simulink model "MPCtest1"  (Simulink 10.1)
settings: Solver=VariableStepAuto  StartTime=0.0  StopTime=30  RelTol=1e-3
libraries: Solver_SF x1, sldrtlib x1, simulink x1
settings Model: Creator=27286  LastModifiedBy=27286
settings DataIOCC: SaveFormat=Dataset  ReturnWorkspaceOutputs=on
settings OptimizationCC: LifeSpan=auto
settings DebuggingCC: UnderspecifiedInitializationDetection=Simplified  MergeDetectMultiDrivingBlocksExec=error  SFUnexpectedBacktrackingDiag=error  SFNoUnconditionalDefaultTransitionDiag=error  SFExecutionAtInitializationDiag=warning  ArithmeticOperatorsInVariantConditions=error
settings HardwareCC: ProdBitPerPointer=64  ProdBitPerSizeT=64  ProdBitPerPtrDiffT=64  ProdLargestAtomicFloat=Float  ProdIntDivRoundTo=Zero  ProdEndianess=LittleEndian  ProdWordSize=64  ProdHWDeviceType=Intel->x86-64 (Windows64)
settings ModelReferenceCC: PropagateSignalLabelsOutOfModel=on
settings SFSimCC: SimUseLocalCustomCode=on  CustomCodeUndefinedFunction=FilterOut
settings RTWCC: RTWUseLocalCustomCode=on
settings CodeAppCC: StateflowObjectComments=off
settings GRTTargetCC: TargetLangStandard=C99 (ISO)  CombineOutputUpdateFcns=on  GRTInterface=off
settings ConfigComp: CovMetricSettings=dwe  CovHtmlReporting=off  CovSaveCumulativeToWorkspaceVar=off  CovSaveSingleToWorkspaceVar=off  CovExternalEMLEnable=on

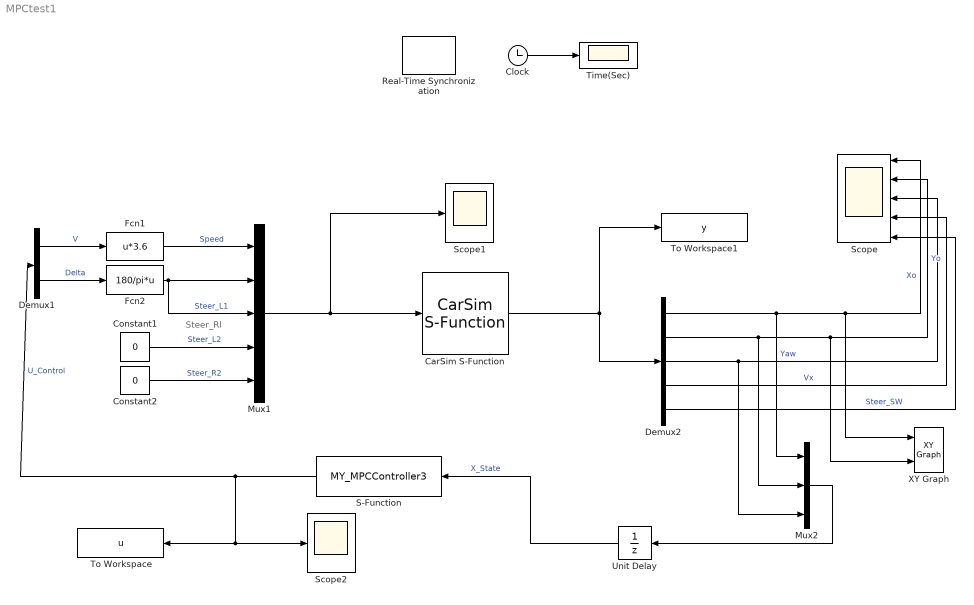
== system MPCtest1 ==
  note: Steer_Rl
  CarSim S-Function : Solver_SF/CarSim S-Function  Priority=1  SIMFILE=simfile.sim  Run_RTs=off  vs_state_ind=Run  StopMode_ind=Vehicle Model
  Clock : Clock
  Constant1 : Constant  Value=0
  Constant2 : Constant  Value=0
  Demux1 : Demux  Outputs=2
  Demux2 : Demux  Outputs=5
  Fcn1 : Fcn  Expr=u*3.6
  Fcn2 : Fcn  Expr=180/pi*u
  Mux1 : Mux  Inputs=5
  Mux2 : Mux  Inputs=3
  Real-Time Synchronization : sldrtlib/Real-Time Synchronization  SampleTime=0.1  MaxMissedTicks=10  ShowMissedTicks=off  YieldWhenWaiting=off
  S-Function : S-Function  FunctionName=MY_MPCController3  SFunctionDeploymentMode=off  EnableBusSupport=off
  Scope : Scope  NumInputPorts=5
  Scope1 : Scope
  Scope2 : Scope
  Time(Sec) : Scope
  To Workspace : ToWorkspace  VariableName=u  SaveFormat=Timeseries  SampleTime=-1
  To Workspace1 : ToWorkspace  VariableName=y  SaveFormat=Timeseries  SampleTime=-1
  Unit Delay : UnitDelay  SampleTime=-1  HasFrameUpgradeWarning=on
  XY Graph : simulink/Sinks/XY Graph  xmin=-50  xmax=50  ymin=0  ymax=100  st=-1
  wires:
  Demux1/2 -> Fcn2/1  "Delta"
  Demux1/1 -> Fcn1/1  "V"
  Fcn1/1 -> Mux1/1  "Speed"
  Constant1/1 -> Mux1/4  "Steer_L2"
  Constant2/1 -> Mux1/5  "Steer_R2"
  Fcn2/1 -> Mux1/3, Mux1/2  "Steer_L1"
  Mux1/1 -> CarSim S-Function/1, Scope1/1
  CarSim S-Function/1 -> Demux2/1, To Workspace1/1
  Demux2/1 -> Mux2/1, XY Graph/1, Scope/1  "Xo"
  Demux2/2 -> Mux2/2, XY Graph/2, Scope/2  "Yo"
  Demux2/3 -> Mux2/3, Scope/3  "Yaw"
  Demux2/4 -> Scope/4  "Vx"
  Demux2/5 -> Scope/5  "Steer_SW"
  Mux2/1 -> Unit Delay/1
  Unit Delay/1 -> S-Function/1  "X_State"
  S-Function/1 -> Scope2/1, To Workspace/1, Demux1/1  "U_Control"
  Clock/1 -> Time(Sec)/1
